simulink model "test_multisrc_coupling"  (R2025b)
settings: Solver=FixedStepAuto  StartTime=0.0  StopTime=5  FixedStep=50e-6  RelTol=1e-3
undefined symbols (not defined in the file or in its folder): D_ES101, D_ES102, delta0_ES101, delta0_ES102, M_ES101, M_ES102, Pe_scale, Pm_ES101, Pm_ES102, Pm_step_amp_ES101, Pm_step_amp_ES102, Pm_step_t_ES101, Pm_step_t_ES102, Vmag_ES101, Vmag_ES102, VSGScale_ES101, VSGScale_ES102, wn_const
libraries: spsControlledVoltageSourceLib x6, spsSeriesRLCBranchLib x6, spsGroundLib x2, spsThreePhasePISectionLineLib x2, spsThreePhaseVIMeasurementLib x2, spsThreePhaseSeriesRLCLoadLib x1, spspowerguiLib x1
settings Model: Creator=27443  LastModifiedBy=27443

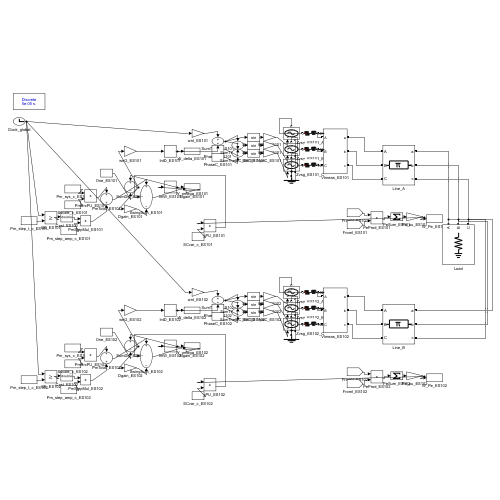
[thumbnail: Simulink's stored preview of the top-level diagram]
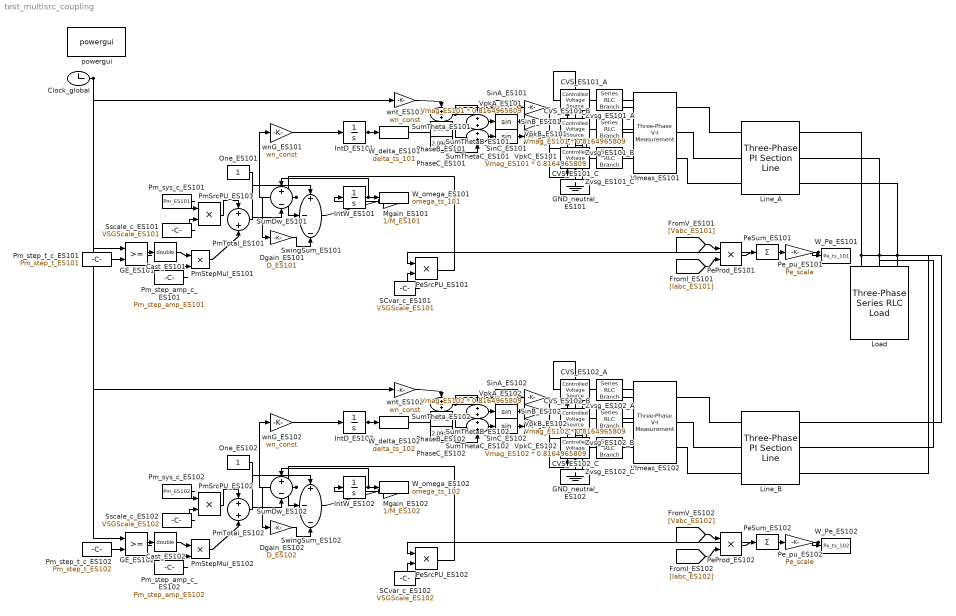
== system test_multisrc_coupling ==
  CVS_ES101_A : spsControlledVoltageSourceLib/Controlled Voltage Source  Initialize=on  Source_Type=AC  Amplitude=0  Phase=0  Frequency=0  Measurements=None
  CVS_ES101_B : spsControlledVoltageSourceLib/Controlled Voltage Source  Initialize=on  Source_Type=AC  Amplitude=0  Phase=0  Frequency=0  Measurements=None
  CVS_ES101_C : spsControlledVoltageSourceLib/Controlled Voltage Source  Initialize=on  Source_Type=AC  Amplitude=0  Phase=0  Frequency=0  Measurements=None
  CVS_ES102_A : spsControlledVoltageSourceLib/Controlled Voltage Source  Initialize=on  Source_Type=AC  Amplitude=0  Phase=0  Frequency=0  Measurements=None
  CVS_ES102_B : spsControlledVoltageSourceLib/Controlled Voltage Source  Initialize=on  Source_Type=AC  Amplitude=0  Phase=0  Frequency=0  Measurements=None
  CVS_ES102_C : spsControlledVoltageSourceLib/Controlled Voltage Source  Initialize=on  Source_Type=AC  Amplitude=0  Phase=0  Frequency=0  Measurements=None
  Cast_ES101 : DataTypeConversion  OutDataTypeStr=double  SaturateOnIntegerOverflow=off  RndMeth=Floor
  Cast_ES102 : DataTypeConversion  OutDataTypeStr=double  SaturateOnIntegerOverflow=off  RndMeth=Floor
  Clock_global : Clock
  Dgain_ES101 : Gain  Gain=D_ES101
  Dgain_ES102 : Gain  Gain=D_ES102
  GE_ES101 : RelationalOperator  OutDataTypeStr=boolean  RndMeth=Simplest  InputSameDT=off
  GE_ES102 : RelationalOperator  OutDataTypeStr=boolean  RndMeth=Simplest  InputSameDT=off
  GND_neutral_ES101 : spsGroundLib/Ground  LConnTagsString=a
  GND_neutral_ES102 : spsGroundLib/Ground  LConnTagsString=a
  IntD_ES101 : Integrator  InitialCondition=delta0_ES101
  IntD_ES102 : Integrator  InitialCondition=delta0_ES102
  IntW_ES101 : Integrator  InitialCondition=1
  IntW_ES102 : Integrator  InitialCondition=1
  Line_A : spsThreePhasePISectionLineLib/Three-Phase PI Section Line  LConnTagsString=a|b|c  RConnTagsString=A|B|C  Length=50  Frequency=50  Resistances=[0.053 0.159]  Inductances=[0.00141 0.00423]  Capacitances=[9e-09 5.4e-09]
  Line_B : spsThreePhasePISectionLineLib/Three-Phase PI Section Line  LConnTagsString=a|b|c  RConnTagsString=A|B|C  Length=50  Frequency=50  Resistances=[0.053 0.159]  Inductances=[0.00141 0.00423]  Capacitances=[9e-09 5.4e-09]
  Load : spsThreePhaseSeriesRLCLoadLib/Three-Phase Series RLC Load  LConnTagsString=A|B|C  Configuration=Y (grounded)  NominalVoltage=230000  Vabc=[1e3 1e3 1e3]  Vabcp=[1e3 1e3 1e3]  NominalFrequency=50  UnbalancedPower=off  ActivePower=80000000  InductivePower=0  CapacitivePower=0  Pabc=[10e3 9e3 11e3]  QLabc=[100 90 110]  QCabc=[100 90 110]  Pabcp=[10e3 9e3 11e3]  QLabcp=[100 90 110]  QCabcp=[100 90 110]  Measurements=None  LoadType=constant Z
  Mgain_ES101 : Gain  Gain=1/M_ES101
  Mgain_ES102 : Gain  Gain=1/M_ES102
  One_ES101 : Constant
  One_ES102 : Constant
  PeProd_ES101 : Product
  PeProd_ES102 : Product
  PeSrcPU_ES101 : Product
  PeSrcPU_ES102 : Product
  PeSum_ES101 : Sum  Inputs=+
  PeSum_ES102 : Sum  Inputs=+
  Pe_pu_ES101 : Gain  Gain=Pe_scale
  Pe_pu_ES102 : Gain  Gain=Pe_scale
  PhaseB_ES101 : Constant  Value=-2.0944
  PhaseB_ES102 : Constant  Value=-2.0944
  PhaseC_ES101 : Constant  Value=2.0944
  PhaseC_ES102 : Constant  Value=2.0944
  PmSrcPU_ES101 : Product
  PmSrcPU_ES102 : Product
  PmStepMul_ES101 : Product
  PmStepMul_ES102 : Product
  PmTotal_ES101 : Sum
  PmTotal_ES102 : Sum
  Pm_step_amp_c_ES101 : Constant  Value=Pm_step_amp_ES101
  Pm_step_amp_c_ES102 : Constant  Value=Pm_step_amp_ES102
  Pm_step_t_c_ES101 : Constant  Value=Pm_step_t_ES101
  Pm_step_t_c_ES102 : Constant  Value=Pm_step_t_ES102
  Pm_sys_c_ES101 : Constant  Value=Pm_ES101
  Pm_sys_c_ES102 : Constant  Value=Pm_ES102
  SCvar_c_ES101 : Constant  Value=VSGScale_ES101
  SCvar_c_ES102 : Constant  Value=VSGScale_ES102
  SinA_ES101 : Trigonometry
  SinA_ES102 : Trigonometry
  SinB_ES101 : Trigonometry
  SinB_ES102 : Trigonometry
  SinC_ES101 : Trigonometry
  SinC_ES102 : Trigonometry
  Sscale_c_ES101 : Constant  Value=VSGScale_ES101
  Sscale_c_ES102 : Constant  Value=VSGScale_ES102
  SumDw_ES101 : Sum  Inputs=+-
  SumDw_ES102 : Sum  Inputs=+-
  SumThetaB_ES101 : Sum
  SumThetaB_ES102 : Sum
  SumThetaC_ES101 : Sum
  SumThetaC_ES102 : Sum
  SumTheta_ES101 : Sum
  SumTheta_ES102 : Sum
  SwingSum_ES101 : Sum  Inputs=+--
  SwingSum_ES102 : Sum  Inputs=+--
  VImeas_ES101 : spsThreePhaseVIMeasurementLib/Three-Phase V-I Measurement  VoltageMeasurement=phase-to-ground  SetLabelV=on  LabelV=Vabc_ES101  Vpu=off  VpuLL=off  CurrentMeasurement=yes  SetLabelI=on  LabelI=Iabc_ES101  Ipu=off  Pbase=100e6  Vbase=500e3  OutputType=Complex  PhasorSimulation=off  PSBequivalent=0
  VImeas_ES102 : spsThreePhaseVIMeasurementLib/Three-Phase V-I Measurement  VoltageMeasurement=phase-to-ground  SetLabelV=on  LabelV=Vabc_ES102  Vpu=off  VpuLL=off  CurrentMeasurement=yes  SetLabelI=on  LabelI=Iabc_ES102  Ipu=off  Pbase=100e6  Vbase=500e3  OutputType=Complex  PhasorSimulation=off  PSBequivalent=0
  VpkA_ES101 : Gain  Gain=Vmag_ES101 * 0.8164965809
  VpkA_ES102 : Gain  Gain=Vmag_ES102 * 0.8164965809
  VpkB_ES101 : Gain  Gain=Vmag_ES101 * 0.8164965809
  VpkB_ES102 : Gain  Gain=Vmag_ES102 * 0.8164965809
  VpkC_ES101 : Gain  Gain=Vmag_ES101 * 0.8164965809
  VpkC_ES102 : Gain  Gain=Vmag_ES102 * 0.8164965809
  W_Pe_ES101 : ToWorkspace  VariableName=Pe_ts_101  SaveFormat=Timeseries  SampleTime=-1
  W_Pe_ES102 : ToWorkspace  VariableName=Pe_ts_102  SaveFormat=Timeseries  SampleTime=-1
  W_delta_ES101 : ToWorkspace  VariableName=delta_ts_101  SaveFormat=Timeseries  SampleTime=-1
      settings: MaxDataPoints=2
  W_delta_ES102 : ToWorkspace  VariableName=delta_ts_102  SaveFormat=Timeseries  SampleTime=-1
      settings: MaxDataPoints=2
  W_omega_ES101 : ToWorkspace  VariableName=omega_ts_101  SaveFormat=Timeseries  SampleTime=-1
  W_omega_ES102 : ToWorkspace  VariableName=omega_ts_102  SaveFormat=Timeseries  SampleTime=-1
  Zvsg_ES101_A : spsSeriesRLCBranchLib/Series RLC Branch  LConnTagsString=__new0  RConnTagsString=__new0  BranchType=RL  Resistance=0.7935  Inductance=0.25258  SetiL0=off  InitialCurrent=0  Capacitance=1e-6  Setx0=off  InitialVoltage=0  Measurements=None
  Zvsg_ES101_B : spsSeriesRLCBranchLib/Series RLC Branch  LConnTagsString=__new0  RConnTagsString=__new0  BranchType=RL  Resistance=0.7935  Inductance=0.25258  SetiL0=off  InitialCurrent=0  Capacitance=1e-6  Setx0=off  InitialVoltage=0  Measurements=None
  Zvsg_ES101_C : spsSeriesRLCBranchLib/Series RLC Branch  LConnTagsString=__new0  RConnTagsString=__new0  BranchType=RL  Resistance=0.7935  Inductance=0.25258  SetiL0=off  InitialCurrent=0  Capacitance=1e-6  Setx0=off  InitialVoltage=0  Measurements=None
  Zvsg_ES102_A : spsSeriesRLCBranchLib/Series RLC Branch  LConnTagsString=__new0  RConnTagsString=__new0  BranchType=RL  Resistance=0.7935  Inductance=0.25258  SetiL0=off  InitialCurrent=0  Capacitance=1e-6  Setx0=off  InitialVoltage=0  Measurements=None
  Zvsg_ES102_B : spsSeriesRLCBranchLib/Series RLC Branch  LConnTagsString=__new0  RConnTagsString=__new0  BranchType=RL  Resistance=0.7935  Inductance=0.25258  SetiL0=off  InitialCurrent=0  Capacitance=1e-6  Setx0=off  InitialVoltage=0  Measurements=None
  Zvsg_ES102_C : spsSeriesRLCBranchLib/Series RLC Branch  LConnTagsString=__new0  RConnTagsString=__new0  BranchType=RL  Resistance=0.7935  Inductance=0.25258  SetiL0=off  InitialCurrent=0  Capacitance=1e-6  Setx0=off  InitialVoltage=0  Measurements=None
  powergui : spspowerguiLib/powergui  Priority=1  SimulationMode=Discrete  SampleTime=50e-6  frequency=60  Iterations=50  frequencyindice=60  Pbase=100e6  ErrMax=1e-4  UnitsV=kV  UnitsW=MW  buscounter=0  FunctionMessages=off  echomessages=off  EnableUseOfTLC=off  CurrentSourceSwitches=off  DisableSnubberDevices=off  DisableRonSwitches=off  DisableVfSwitches=off  DisplayEquations=off  AutomaticDiscreteSolvers=off  SolverType=Tustin/Backward Euler (TBE)  Interpol=off  ExternalGateDelay=off  methode=off  Ts=100  x0status=blocks  SPID=on  SwTol=0  HookPort=off  NonlinearTolerance=1e-4  nMaxIteration=100  ContinueOnMaxIteration=off  RestoreLinks=warning  ResistiveCurrentMeasurement=off  Frange=[0:2:500]  Ylog=off  Xlog=on  ShowGrid=off  save=off  variable=ZData  structure=0  ZoomFFT=off  StartTime=0.0  cycles=1  DisplayStyle=1  fundamental=60  FreqAxis=off  MaxFrequency=1000  frequencyindicesteady=1  RmsSteady=1  display=off
  wnG_ES101 : Gain  Gain=wn_const
  wnG_ES102 : Gain  Gain=wn_const
  wnt_ES101 : Gain  Gain=wn_const
  wnt_ES102 : Gain  Gain=wn_const
  wires:
  Clock_global/1 -> GE_ES101/1, wnt_ES101/1, GE_ES102/1, wnt_ES102/1
  Pm_step_t_c_ES101/1 -> GE_ES101/2
  GE_ES101/1 -> Cast_ES101/1
  Cast_ES101/1 -> PmStepMul_ES101/1
  Pm_step_amp_c_ES101/1 -> PmStepMul_ES101/2
  Pm_sys_c_ES101/1 -> PmSrcPU_ES101/1
  Sscale_c_ES101/1 -> PmSrcPU_ES101/2
  PmSrcPU_ES101/1 -> PmTotal_ES101/1
  PmStepMul_ES101/1 -> PmTotal_ES101/2
  IntW_ES101/1 -> SumDw_ES101/1, W_omega_ES101/1
  One_ES101/1 -> SumDw_ES101/2
  SumDw_ES101/1 -> Dgain_ES101/1, wnG_ES101/1
  PmTotal_ES101/1 -> SwingSum_ES101/1
  Dgain_ES101/1 -> SwingSum_ES101/3
  SwingSum_ES101/1 -> Mgain_ES101/1
  Mgain_ES101/1 -> IntW_ES101/1
  wnG_ES101/1 -> IntD_ES101/1
  wnt_ES101/1 -> SumTheta_ES101/1
  IntD_ES101/1 -> SumTheta_ES101/2, W_delta_ES101/1
  SumTheta_ES101/1 -> SumThetaB_ES101/1, SumThetaC_ES101/1, SinA_ES101/1
  PhaseB_ES101/1 -> SumThetaB_ES101/2
  PhaseC_ES101/1 -> SumThetaC_ES101/2
  SumThetaB_ES101/1 -> SinB_ES101/1
  SumThetaC_ES101/1 -> SinC_ES101/1
  SinA_ES101/1 -> VpkA_ES101/1
  SinB_ES101/1 -> VpkB_ES101/1
  SinC_ES101/1 -> VpkC_ES101/1
  VpkA_ES101/1 -> CVS_ES101_A/1
  VpkB_ES101/1 -> CVS_ES101_B/1
  VpkC_ES101/1 -> CVS_ES101_C/1
  [Vabc_ES101] -> PeProd_ES101/1
  [Iabc_ES101] -> PeProd_ES101/2
  PeProd_ES101/1 -> PeSum_ES101/1
  PeSum_ES101/1 -> Pe_pu_ES101/1
  Pe_pu_ES101/1 -> PeSrcPU_ES101/1, W_Pe_ES101/1
  SCvar_c_ES101/1 -> PeSrcPU_ES101/2
  PeSrcPU_ES101/1 -> SwingSum_ES101/2
  Pm_step_t_c_ES102/1 -> GE_ES102/2
  GE_ES102/1 -> Cast_ES102/1
  Cast_ES102/1 -> PmStepMul_ES102/1
  Pm_step_amp_c_ES102/1 -> PmStepMul_ES102/2
  Pm_sys_c_ES102/1 -> PmSrcPU_ES102/1
  Sscale_c_ES102/1 -> PmSrcPU_ES102/2
  PmSrcPU_ES102/1 -> PmTotal_ES102/1
  PmStepMul_ES102/1 -> PmTotal_ES102/2
  IntW_ES102/1 -> SumDw_ES102/1, W_omega_ES102/1
  One_ES102/1 -> SumDw_ES102/2
  SumDw_ES102/1 -> Dgain_ES102/1, wnG_ES102/1
  PmTotal_ES102/1 -> SwingSum_ES102/1
  Dgain_ES102/1 -> SwingSum_ES102/3
  SwingSum_ES102/1 -> Mgain_ES102/1
  Mgain_ES102/1 -> IntW_ES102/1
  wnG_ES102/1 -> IntD_ES102/1
  wnt_ES102/1 -> SumTheta_ES102/1
  IntD_ES102/1 -> SumTheta_ES102/2, W_delta_ES102/1
  SumTheta_ES102/1 -> SumThetaB_ES102/1, SumThetaC_ES102/1, SinA_ES102/1
  PhaseB_ES102/1 -> SumThetaB_ES102/2
  PhaseC_ES102/1 -> SumThetaC_ES102/2
  SumThetaB_ES102/1 -> SinB_ES102/1
  SumThetaC_ES102/1 -> SinC_ES102/1
  SinA_ES102/1 -> VpkA_ES102/1
  SinB_ES102/1 -> VpkB_ES102/1
  SinC_ES102/1 -> VpkC_ES102/1
  VpkA_ES102/1 -> CVS_ES102_A/1
  VpkB_ES102/1 -> CVS_ES102_B/1
  VpkC_ES102/1 -> CVS_ES102_C/1
  [Vabc_ES102] -> PeProd_ES102/1
  [Iabc_ES102] -> PeProd_ES102/2
  PeProd_ES102/1 -> PeSum_ES102/1
  PeSum_ES102/1 -> Pe_pu_ES102/1
  Pe_pu_ES102/1 -> PeSrcPU_ES102/1, W_Pe_ES102/1
  SCvar_c_ES102/1 -> PeSrcPU_ES102/2
  PeSrcPU_ES102/1 -> SwingSum_ES102/2
  connections:
  CVS_ES101_A/LConn1 -- CVS_ES101_B/LConn1 -- GND_neutral_ES101/LConn1 -- CVS_ES101_C/LConn1
  CVS_ES101_A/RConn1 -- Zvsg_ES101_A/LConn1
  CVS_ES101_B/RConn1 -- Zvsg_ES101_B/LConn1
  CVS_ES101_C/RConn1 -- Zvsg_ES101_C/LConn1
  Zvsg_ES101_A/RConn1 -- VImeas_ES101/LConn1
  Zvsg_ES101_B/RConn1 -- VImeas_ES101/LConn2
  Zvsg_ES101_C/RConn1 -- VImeas_ES101/LConn3
  CVS_ES102_A/LConn1 -- CVS_ES102_B/LConn1 -- GND_neutral_ES102/LConn1 -- CVS_ES102_C/LConn1
  CVS_ES102_A/RConn1 -- Zvsg_ES102_A/LConn1
  CVS_ES102_B/RConn1 -- Zvsg_ES102_B/LConn1
  CVS_ES102_C/RConn1 -- Zvsg_ES102_C/LConn1
  Zvsg_ES102_A/RConn1 -- VImeas_ES102/LConn1
  Zvsg_ES102_B/RConn1 -- VImeas_ES102/LConn2
  Zvsg_ES102_C/RConn1 -- VImeas_ES102/LConn3
  VImeas_ES101/RConn1 -- Line_A/LConn1
  VImeas_ES101/RConn2 -- Line_A/LConn2
  VImeas_ES101/RConn3 -- Line_A/LConn3
  VImeas_ES102/RConn1 -- Line_B/LConn1
  VImeas_ES102/RConn2 -- Line_B/LConn2
  VImeas_ES102/RConn3 -- Line_B/LConn3
  Load/LConn1 -- Line_A/RConn1 -- Line_B/RConn1
  Load/LConn2 -- Line_A/RConn2 -- Line_B/RConn2
  Load/LConn3 -- Line_A/RConn3 -- Line_B/RConn3
